simulink model "TemperatureModel"  (R2021a)
settings: Solver=VariableStepAuto  StartTime=0.0  StopTime=10.0  RelTol=1e-3
InitFcn:
  | readTelemetry
libraries: vrlib x1
settings Model: Creator=0170469501  LastModifiedBy=0170469501
settings DataIOCC: ReturnWorkspaceOutputs=off

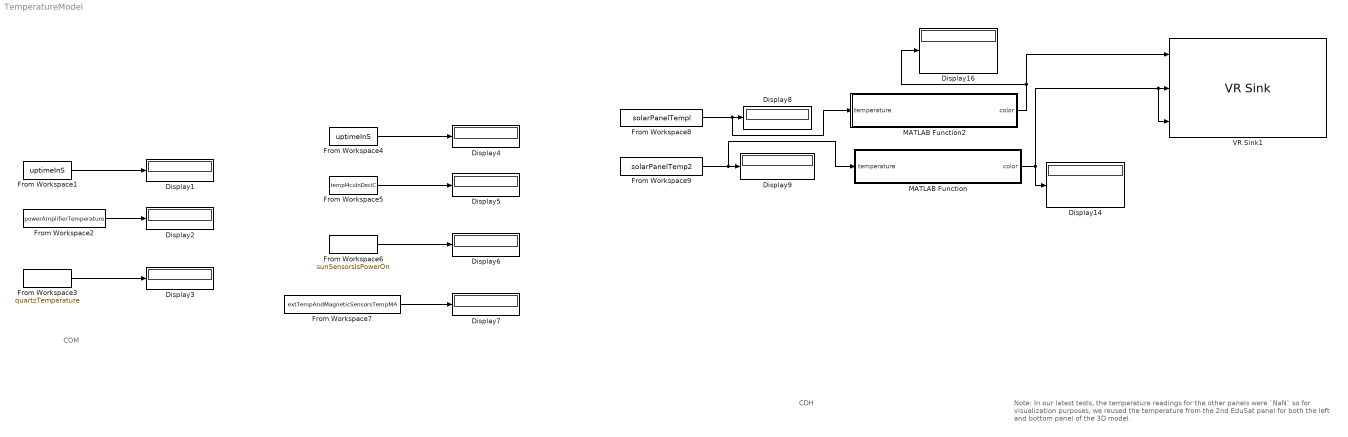
== system TemperatureModel ==
  note: COM
  note: CDH
  note: Note: In our latest tests, the temperature readings for the other panels were `NaN` so for visualization purposes, we reused the temperature from the 2nd EduSat panel for both the left and bottom panel of the 3D model.
  Display{1..9,14,16} (11 alike) : Display
  From Workspace1 : FromWorkspace  VariableName=uptimeInS
  From Workspace2 : FromWorkspace  VariableName=powerAmplifierTemperature
  From Workspace3 : FromWorkspace  VariableName=quartzTemperature
  From Workspace4 : FromWorkspace  VariableName=uptimeInS
  From Workspace5 : FromWorkspace  VariableName=templ4cuInDeciC
  From Workspace6 : FromWorkspace  VariableName=sunSensorsIsPowerOn
  From Workspace7 : FromWorkspace  VariableName=extTempAndMagneticSensorsTempMA
  From Workspace8 : FromWorkspace  VariableName=solarPanelTempl
  From Workspace9 : FromWorkspace  VariableName=solarPanelTemp2
  MATLAB Function : MATLAB Function  TreatAsAtomicUnit=on
  MATLAB Function2 : MATLAB Function  TreatAsAtomicUnit=on
  VR Sink1 : vrlib/VR Sink  InstantiateOnLoad=on  SampleTime=0.1  ViewEnable=on  RemoteChange=off  RemoteView=off  FieldsWritten=right_panel_material.diffuseColor.3.1.1.double#left_panel_material.diffuseColor.3.1.1.double#bottom_panel_material.diffuseColor.3.1.1.double  WorldFileName=sat_virtual_world.x3d  AutoView=on  VideoDimensions=[]  AllowVariableSize=off  FigureProperties="{'Position', 'Name', 'Viewpoint', 'CameraBound', 'CameraDirection', 'CameraPosition', 'CameraUpVector', 'ZoomFactor', 'Antialiasing', 'Headlight', 'Lighting', 'NavPanel', 'Sound', 'StatusBar', 'Stereo3D', 'Stereo3DCameraOffset', 'Stereo3DHIT', 'ToolBar', 'Textures', 'Transparency', 'Triad', 'Wireframe', 'NavZones', 'NavMode', 'NavSpeed', 'CaptureFileFormat', 'CaptureFileName', 'Record2DCompressMethod', 'Record2DCompressQuality', 'Record2D', 'Record2DFileName', 'Record2DFPS'; [5.0000000000000000e+00   9.2000000000000000e+01   5.7600000000000000e+02   3.5000000000000000e+02], '', '', 'on', [-3.6939445387069053e-01   0.0000000000000000e+00  -9.2927269272779900e-01], [1.0713395706918615e+01   3.7993745803833008e+00   3.6951314435034163e+01], [0.0000000000000000e+00   1.0000000000000000e+00   0.0000000000000000e+00], [1.0000000000000000e+00], 'on', 'on', 'on', 'halfbar', 'on', 'on', 'off', [1.0000000149011612e-01], [0.0000000000000000e+00], 'on', 'on', 'on', 'none', 'off', 'off', 'fly', 'normal', 'tif', '%f_anim_%n.tif', 'auto', [7.5000000000000000e+01], 'off', '%f_anim_%n.avi', 'auto'}"
  wires:
  From Workspace1/1 -> Display1/1
  From Workspace2/1 -> Display2/1
  From Workspace3/1 -> Display3/1
  From Workspace5/1 -> Display5/1
  From Workspace4/1 -> Display4/1
  From Workspace6/1 -> Display6/1
  From Workspace8/1 -> MATLAB Function2/1(temperature), Display8/1
  From Workspace7/1 -> Display7/1
  From Workspace9/1 -> MATLAB Function/1(temperature), Display9/1
  MATLAB Function/1(color) -> Display14/1, VR Sink1/3, VR Sink1/2
  MATLAB Function2/1(color) -> VR Sink1/1, Display16/1

== matlab function TemperatureModel/MATLAB Function2 ==
  data: temperature input; color output
function color  = getTemperatureColor(temperature)
    if (temperature <= 30)
        disp(temperature)
        color = [0.2, 0.8, 1.0];
    else
        disp(temperature)
        color = [1.0, 0.2, 0.2];
    end
end

== matlab function TemperatureModel/MATLAB Function ==
  data: temperature input; color output
function color  = getTemperatureColor(temperature)
    if (temperature <= 30)
        disp(temperature)
        color = [0.2, 0.8, 1.0];
    else
        disp(temperature)
        color = [1.0, 0.2, 0.2];
    end
end
